simulink model "BLOC_LithiumIon_Battery_Management_System"  (R2016a)
settings: Solver=VariableStepAuto  StartTime=0.0  StopTime=10.0  RelTol=1e-3
undefined symbols (not defined in the file): DiscIntNeverNeededParam, hev_dt, syse_bat_nominal_capacity_as, syse_cdl, syse_max_charge_current, syse_max_discharge_current, syse_nb_cell, syse_rdl, syse_rser, syse_soc_current_limits, syse_soc_initial, syse_soc_ocv, syse_vocv
settings Model: Creator=Florent  LastModifiedBy=Florent

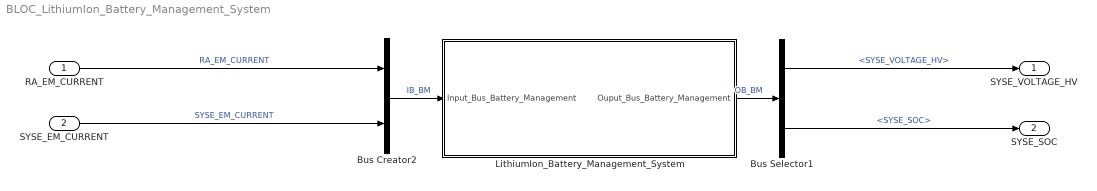
== system BLOC_LithiumIon_Battery_Management_System ==
  RA_EM_CURRENT : Inport
  SYSE_EM_CURRENT : Inport  Port=2
  Bus Creator2 : BusCreator  Inputs=2
  Bus Selector1 : BusSelector  OutputSignals=SYSE_VOLTAGE_HV,SYSE_SOC
  LithiumIon_Battery_Management_System : Subsystem  TreatAsAtomicUnit=on  SystemSampleTime=hev_dt
  SYSE_VOLTAGE_HV : Outport
  SYSE_SOC : Outport  Port=2
  wires:
  Bus Selector1/2 -> SYSE_SOC/1  "<SYSE_SOC>"
  Bus Selector1/1 -> SYSE_VOLTAGE_HV/1  "<SYSE_VOLTAGE_HV>"
  RA_EM_CURRENT/1 -> Bus Creator2/1  "RA_EM_CURRENT"
  SYSE_EM_CURRENT/1 -> Bus Creator2/2  "SYSE_EM_CURRENT"
  Bus Creator2/1 -> LithiumIon_Battery_Management_System/1("Input_Bus_Battery_Management ")  "IB_BM"
  LithiumIon_Battery_Management_System/1(Ouput_Bus_Battery_Management) -> Bus Selector1/1  "OB_BM"

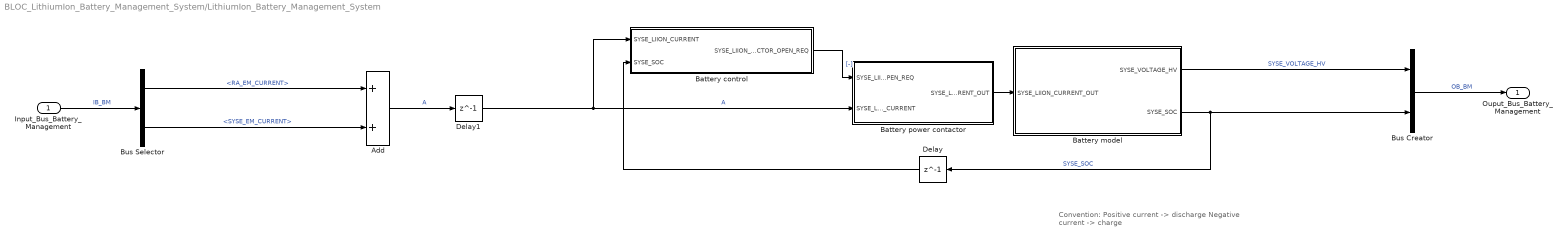
== system BLOC_LithiumIon_Battery_Management_System/LithiumIon_Battery_Management_System ==
  note: Convention:
      | Positive current -> discharge
      | Negative current -> charge
  "Input_Bus_Battery_Management " : Inport
  Add : Sum  SampleTime=hev_dt
  Battery control : Subsystem
  Battery model : Subsystem
  Battery power contactor : Subsystem
  Bus Creator : BusCreator  Inputs=2
  Bus Selector : BusSelector  OutputSignals=RA_EM_CURRENT,SYSE_EM_CURRENT
  Delay : Delay  DelayLength=1  SampleTime=hev_dt
  Delay1 : Delay  DelayLength=1  SampleTime=hev_dt
  Ouput_Bus_Battery_Management : Outport
  wires:
  Delay1/1 -> Battery control/1(SYSE_LIION_CURRENT), Battery power contactor/2(SYSE_LIION_CURRENT)  "A"
  Battery model/2(SYSE_SOC) -> Delay/1, Bus Creator/2  "SYSE_SOC"
  Battery model/1(SYSE_VOLTAGE_HV) -> Bus Creator/1  "SYSE_VOLTAGE_HV"
  Battery control/1(SYSE_LIION_CONTACTOR_OPEN_REQ) -> Battery power contactor/1(SYSE_LIION_CONTACTOR_OPEN_REQ)  "[-]"
  Battery power contactor/1(SYSE_LIION_CURRENT_OUT) -> Battery model/1(SYSE_LIION_CURRENT_OUT)
  Delay/1 -> Battery control/2(SYSE_SOC)
  Add/1 -> Delay1/1  "A"
  "Input_Bus_Battery_Management "/1 -> Bus Selector/1  "IB_BM"
  Bus Selector/2 -> Add/2  "<SYSE_EM_CURRENT>"
  Bus Selector/1 -> Add/1  "<RA_EM_CURRENT>"
  Bus Creator/1 -> Ouput_Bus_Battery_Management/1  "OB_BM"

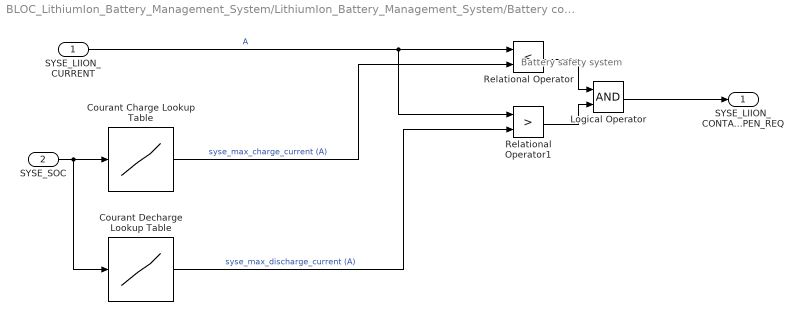
== system BLOC_LithiumIon_Battery_Management_System/LithiumIon_Battery_Management_System/Battery control ==
  note: Battery safety system
  SYSE_LIION_CURRENT : Inport
  SYSE_SOC : Inport  Port=2
  Courant Charge Lookup Table : Lookup_n-D  NumberOfTableDimensions=1  BreakpointsForDimension1=syse_soc_current_limits/100  Table=-syse_max_charge_current  SampleTime=hev_dt  RndMeth=Simplest  InputSameDT=on
  Courant Decharge Lookup Table : Lookup_n-D  NumberOfTableDimensions=1  BreakpointsForDimension1=syse_soc_current_limits/100  Table=syse_max_discharge_current  SampleTime=hev_dt  RndMeth=Simplest  InputSameDT=on
  Logical Operator : Logic  AllPortsSameDT=off  OutDataTypeStr=boolean  SampleTime=hev_dt
  Relational Operator : RelationalOperator  Operator=<  OutDataTypeStr=boolean  SampleTime=hev_dt
  Relational Operator1 : RelationalOperator  Operator=>  OutDataTypeStr=boolean  SampleTime=hev_dt
  SYSE_LIION_CONTACTOR_OPEN_REQ : Outport
  wires:
  SYSE_LIION_CURRENT/1 -> Relational Operator/1, Relational Operator1/1  "A"
  Courant Charge Lookup Table/1 -> Relational Operator/2  "syse_max_charge_current (A)"
  Courant Decharge Lookup Table/1 -> Relational Operator1/2  "syse_max_discharge_current (A)"
  SYSE_SOC/1 -> Courant Charge Lookup Table/1, Courant Decharge Lookup Table/1
  Logical Operator/1 -> SYSE_LIION_CONTACTOR_OPEN_REQ/1
  Relational Operator/1 -> Logical Operator/1
  Relational Operator1/1 -> Logical Operator/2

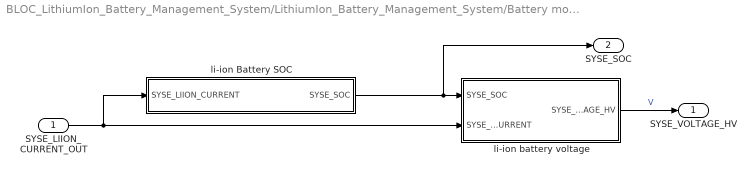
== system BLOC_LithiumIon_Battery_Management_System/LithiumIon_Battery_Management_System/Battery model ==
  SYSE_LIION_CURRENT_OUT : Inport
  li-ion Battery SOC : Subsystem
  li-ion battery voltage : Subsystem
  SYSE_VOLTAGE_HV : Outport
  SYSE_SOC : Outport  Port=2
  wires:
  li-ion battery voltage/1(SYSE_VOLTAGE_HV) -> SYSE_VOLTAGE_HV/1  "V"
  SYSE_LIION_CURRENT_OUT/1 -> li-ion Battery SOC/1(SYSE_LIION_CURRENT), li-ion battery voltage/2(SYSE_LIION_CURRENT)
  li-ion Battery SOC/1(SYSE_SOC) -> li-ion battery voltage/1(SYSE_SOC), SYSE_SOC/1

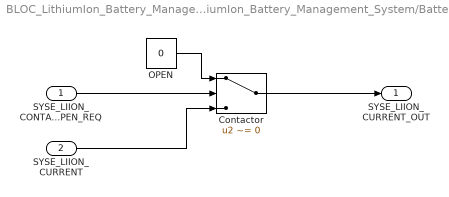
== system BLOC_LithiumIon_Battery_Management_System/LithiumIon_Battery_Management_System/Battery power contactor ==
  SYSE_LIION_CONTACTOR_OPEN_REQ : Inport
  SYSE_LIION_CURRENT : Inport  Port=2
  Contactor : Switch  Criteria=u2 ~= 0  SampleTime=hev_dt
  OPEN : Constant  Value=0
  SYSE_LIION_CURRENT_OUT : Outport
  wires:
  OPEN/1 -> Contactor/1
  SYSE_LIION_CURRENT/1 -> Contactor/3
  SYSE_LIION_CONTACTOR_OPEN_REQ/1 -> Contactor/2
  Contactor/1 -> SYSE_LIION_CURRENT_OUT/1

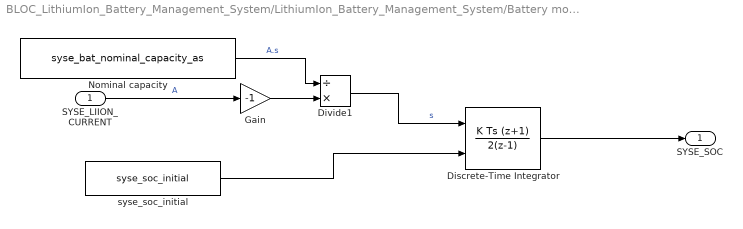
== system BLOC_LithiumIon_Battery_Management_System/LithiumIon_Battery_Management_System/Battery model/li-ion Battery SOC ==
  SYSE_LIION_CURRENT : Inport
  Discrete-Time Integrator : DiscreteIntegrator  IntegratorMethod=Integration: Trapezoidal  InitialConditionSource=external  SampleTime=hev_dt  LimitOutput=on  UpperSaturationLimit=1  LowerSaturationLimit=0  ICPrevOutput=DiscIntNeverNeededParam  ICPrevScaledInput=DiscIntNeverNeededParam
  Divide1 : Product  Inputs=/*  SampleTime=hev_dt
  Gain : Gain  Gain=-1  SampleTime=hev_dt
  Nominal capacity : Constant  Value=syse_bat_nominal_capacity_as
  syse_soc_initial : Constant  Value=syse_soc_initial
  SYSE_SOC : Outport
  wires:
  Nominal capacity/1 -> Divide1/1  "A.s"
  Discrete-Time Integrator/1 -> SYSE_SOC/1
  syse_soc_initial/1 -> Discrete-Time Integrator/2
  Divide1/1 -> Discrete-Time Integrator/1  "s"
  SYSE_LIION_CURRENT/1 -> Gain/1  "A"
  Gain/1 -> Divide1/2

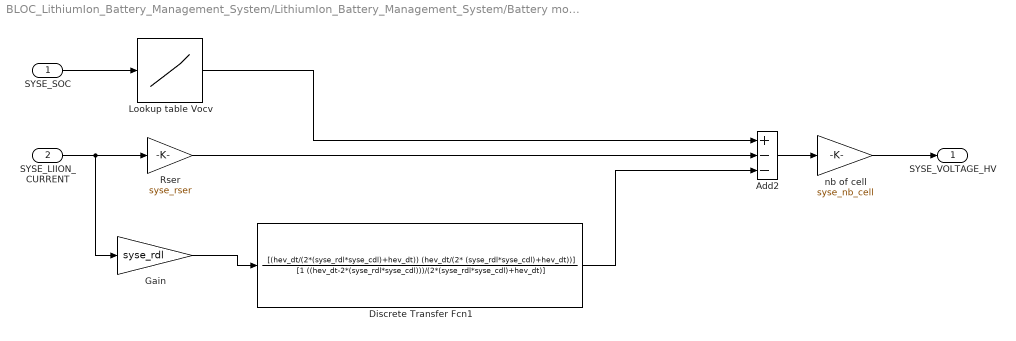
== system BLOC_LithiumIon_Battery_Management_System/LithiumIon_Battery_Management_System/Battery model/li-ion battery voltage ==
  SYSE_SOC : Inport
  SYSE_LIION_CURRENT : Inport  Port=2
  Add2 : Sum  Inputs=+--  SampleTime=hev_dt
  Discrete Transfer Fcn1 : DiscreteTransferFcn  Numerator=[(hev_dt/(2*(syse_rdl*syse_cdl)+hev_dt)) (hev_dt/(2* (syse_rdl*syse_cdl)+hev_dt))]  Denominator=[1 ((hev_dt-2*(syse_rdl*syse_cdl)))/(2*(syse_rdl*syse_cdl)+hev_dt)]  SampleTime=hev_dt
  Gain : Gain  Gain=syse_rdl  SampleTime=hev_dt
  Lookup table Vocv : Lookup_n-D  NumberOfTableDimensions=1  BreakpointsForDimension1=syse_soc_ocv/100  Table=syse_vocv  SampleTime=hev_dt  RndMeth=Simplest  InputSameDT=on
  Rser : Gain  Gain=syse_rser  SampleTime=hev_dt
  nb of cell : Gain  Gain=syse_nb_cell  SampleTime=hev_dt
  SYSE_VOLTAGE_HV : Outport
  wires:
  SYSE_LIION_CURRENT/1 -> Gain/1, Rser/1
  SYSE_SOC/1 -> Lookup table Vocv/1
  Lookup table Vocv/1 -> Add2/1
  Add2/1 -> nb of cell/1
  nb of cell/1 -> SYSE_VOLTAGE_HV/1
  Rser/1 -> Add2/2
  Discrete Transfer Fcn1/1 -> Add2/3
  Gain/1 -> Discrete Transfer Fcn1/1
